simulink model "Sensor_IMU"  (R2016b)
settings: Solver=FixedStepAuto  StartTime=0.0  StopTime=10.0  RelTol=1e-3
model workspace (MATLAB code in the model file):
  | wsHandle = get_param(bdroot, 'modelWorkspace');
  | wsHandle.assignin('sens', AC.Sensors.IMU);
libraries: Sensors_Lib x4
settings Model: ParameterArgumentNames=sens  Creator=rega0051  LastModifiedBy=rega0051

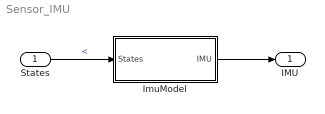
== system Sensor_IMU ==
  "States " : Inport  OutDataTypeStr=Bus: States
  ImuModel : Subsystem  Variant=on
  " IMU" : Outport  OutDataTypeStr=Bus: IMU
  wires:
  "States "/1 -> ImuModel/1(States)  "<"
  ImuModel/1(IMU) -> " IMU"/1

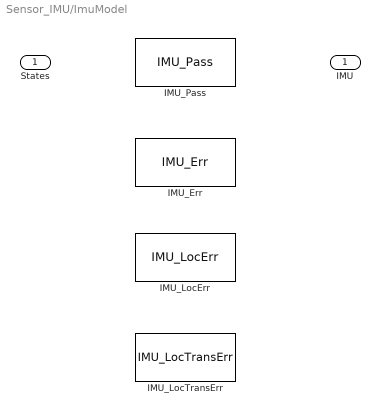
== system Sensor_IMU/ImuModel ==
  States : Inport  OutDataTypeStr=Bus: States
  IMU_Err : Sensors_Lib/IMU Sensor Models/IMU_Err  VariantControl=VarImu_Err
      settings: AttributesFormatString=Variant: %<VariantControl> : %<Variant>
  IMU_LocErr : Sensors_Lib/IMU Sensor Models/IMU_LocErr  VariantControl=VarImu_LocErr
      settings: AttributesFormatString=Variant: %<VariantControl> : %<Variant>
  IMU_LocTransErr : Sensors_Lib/IMU Sensor Models/IMU_LocTransErr  VariantControl=VarImu_LocTransErr
      settings: AttributesFormatString=Variant: %<VariantControl> : %<Variant>
  IMU_Pass : Sensors_Lib/IMU Sensor Models/IMU_Pass  VariantControl=VarImu_Pass
      settings: AttributesFormatString=Variant: %<VariantControl> : %<Variant>
  IMU : Outport  OutDataTypeStr=Bus: IMU
